simulink model "dft_blocks"  (R2018a)
settings: Solver=VariableStepAuto  StartTime=0.0  StopTime=10.0  RelTol=1e-3
settings Model: Creator=berke  LastModifiedBy=berke

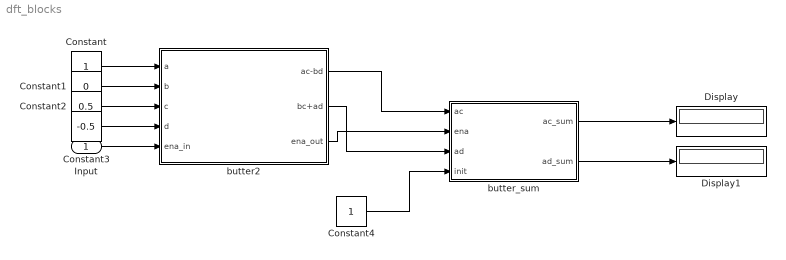
== system dft_blocks ==
  Input : Inport  OutDataTypeStr=boolean  SampleTime=0.1
  Constant : Constant  OutDataTypeStr=fixdt(0,12,0)  SampleTime=0.1
  Constant1 : Constant  Value=0  OutDataTypeStr=fixdt(0,12,0)  SampleTime=0.1
  Constant2 : Constant  Value=0.5  OutDataTypeStr=fixdt(1,16,15)  SampleTime=0.1
  Constant3 : Constant  Value=-0.5  OutDataTypeStr=fixdt(1,16,15)  SampleTime=0.1
  Constant4 : Constant  OutDataTypeStr=boolean  SampleTime=0.1
  Display : Display
  Display1 : Display
  butter2 : Subsystem
  butter_sum : Subsystem
  wires:
  Constant/1 -> butter2/1(a)
  Input/1 -> butter2/5(ena_in)
  Constant3/1 -> butter2/4(d)
  Constant2/1 -> butter2/3(c)
  Constant1/1 -> butter2/2(b)
  butter2/3(ena_out) -> butter_sum/2(ena)
  butter2/1(ac-bd) -> butter_sum/1(ac)
  butter2/2(bc+ad) -> butter_sum/3(ad)
  butter_sum/1(ac_sum) -> Display/1
  butter_sum/2(ad_sum) -> Display1/1
  Constant4/1 -> butter_sum/4(init)

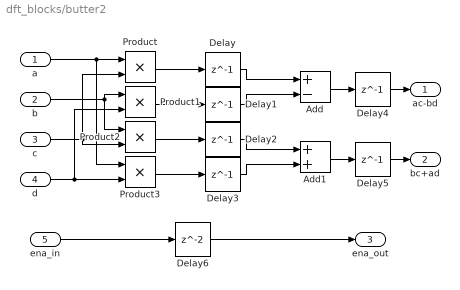
== system dft_blocks/butter2 ==
  a : Inport
  b : Inport  Port=2
  c : Inport  Port=3
  d : Inport  Port=4
  ena_in : Inport  Port=5
  Add : Sum  Inputs=+-
  Add1 : Sum
  Delay{,1..5} (6 alike) : Delay  DelayLength=1
  Delay6 : Delay
  Product{,1..3} (4 alike) : Product
  ac-bd : Outport
  bc+ad : Outport  Port=2
  ena_out : Outport  Port=3
  wires:
  Product2/1 -> Delay2/1
  Delay1/1 -> Add/2
  Delay5/1 -> bc+ad/1
  Delay4/1 -> ac-bd/1
  Product3/1 -> Delay3/1
  Delay3/1 -> Add1/2
  Add1/1 -> Delay5/1
  Product/1 -> Delay/1
  Delay2/1 -> Add1/1
  Product1/1 -> Delay1/1
  a/1 -> Product3/1, Product/1
  Delay/1 -> Add/1
  Add/1 -> Delay4/1
  c/1 -> Product2/2, Product/2
  d/1 -> Product1/2, Product3/2
  b/1 -> Product1/1, Product2/1
  ena_in/1 -> Delay6/1
  Delay6/1 -> ena_out/1

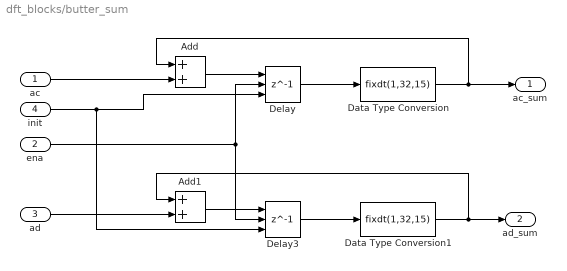
== system dft_blocks/butter_sum ==
  ac : Inport
  ena : Inport  Port=2
  ad : Inport  Port=3
  init : Inport  Port=4
  Add : Sum
  Add1 : Sum
  Data Type Conversion : DataTypeConversion  OutDataTypeStr=fixdt(1,32,15)
  Data Type Conversion1 : DataTypeConversion  OutDataTypeStr=fixdt(1,32,15)
  Delay : Delay  DelayLength=1  ExternalReset=Level  ShowEnablePort=on  SampleTime=0.1
      settings: InputPortMap=u0,e6,r5
  Delay3 : Delay  DelayLength=1  ExternalReset=Level  ShowEnablePort=on  SampleTime=0.1
      settings: InputPortMap=u0,e6,r5
  ac_sum : Outport
  ad_sum : Outport  Port=2
  wires:
  Add/1 -> Delay/1
  ac/1 -> Add/2
  Delay/1 -> Data Type Conversion/1
  Data Type Conversion/1 -> Add/1, ac_sum/1
  ad/1 -> Add1/2
  Delay3/1 -> Data Type Conversion1/1
  Add1/1 -> Delay3/1
  Data Type Conversion1/1 -> ad_sum/1, Add1/1
  ena/1 -> Delay/2, Delay3/2
  init/1 -> Delay3/3, Delay/3
